simulink model "FSAC2021"  (R2014a)
settings: Solver=FixedStepDiscrete  StartTime=0.0  StopTime=inf  FixedStep=0.0005  RelTol=1e-3
model workspace (MAT data in the model file):
  MCOS : class17 (value not decoded)
  MCOS : class17 (value not decoded)
  MCOS : class17 (value not decoded)
  MCOS : class17 (value not decoded)
  MCOS : class17 (value not decoded)
  MCOS : class17 (value not decoded)
  MCOS : class17 (value not decoded)
  MCOS : class17 (value not decoded)
  MCOS : class17 (value not decoded)
  MCOS : class17 (value not decoded)
  MCOS : class17 (value not decoded)
  MCOS : class17 (value not decoded)
  MCOS : class17 (value not decoded)
  MCOS : class17 (value not decoded)
  MCOS : class17 (value not decoded)
  MCOS : class17 (value not decoded)
  MCOS : class17 (value not decoded)
  MCOS : class17 (value not decoded)
  MCOS : class17 (value not decoded)
  BUZZER_START = 1
  MCOS : class17 (value not decoded)
  MCOS : class17 (value not decoded)
  MCOS : class17 (value not decoded)
  MCOS : class17 (value not decoded)
  MCOS : class17 (value not decoded)
  MCOS : class17 (value not decoded)
  MCOS : class17 (value not decoded)
  MCOS : class17 (value not decoded)
  MCOS : class17 (value not decoded)
  MCOS : class17 (value not decoded)
  MCOS : class17 (value not decoded)
  MCOS : class17 (value not decoded)
  MCOS : class17 (value not decoded)
  MCOS : class17 (value not decoded)
  MCOS : class17 (value not decoded)
  MCOS : class17 (value not decoded)
  MCOS : class17 (value not decoded)
  MCOS : class17 (value not decoded)
  MCOS : class17 (value not decoded)
  MCOS : class17 (value not decoded)
  MCOS : class17 (value not decoded)
  MCOS : class17 (value not decoded)
  MCOS : class17 (value not decoded)
  MCOS : class17 (value not decoded)
  MCOS : class17 (value not decoded)
  MCOS : class17 (value not decoded)
  MCOS : class17 (value not decoded)
  MCOS : class17 (value not decoded)
  MCOS : class17 (value not decoded)
  MCOS : class17 (value not decoded)
  MCOS : class17 (value not decoded)
  MCOS : class17 (value not decoded)
  MCOS : class17 (value not decoded)
  MCOS : class17 (value not decoded)
  MCOS : class17 (value not decoded)
  MCOS : class17 (value not decoded)
  MCOS : class17 (value not decoded)
  MCOS : class17 (value not decoded)
  Brake = 11
  MCOS : class17 (value not decoded)
  MCOS : class17 (value not decoded)
  MCOS : class17 (value not decoded)
  MCOS : class17 (value not decoded)
  MCOS : class17 (value not decoded)
  MCOS : class17 (value not decoded)
  MCOS : class17 (value not decoded)
  MCOS : class17 (value not decoded)
  Sensor_Acc_b = 101.85
  Sensor_Acc_k = -0.0185
  Str_Sen_Orig_Angle = -341
  MCOS : class17 (value not decoded)
  Tire_D = 0.47
  T = 0.05
libraries: simulink x396, ec55xxlib x126
(part 13 of 17)

== system FSAC2021/ROUTING/TO_DCAN/Subsystem/DIAG_BCU/Brake_encoder_fault_sts ==
  Brake_encoder_fault_sts : Inport
  Brake_encoder_fault_stsRon : Rounding  Operator=round
  Brake_encoder_fault_sts_1sat : Saturate  UpperLimit=64  LowerLimit=0
  Brake_encoder_fault_sts_Convert : DataTypeConversion  OutDataTypeStr=uint8
  Brake_encoder_fault_sts_Convert1 : DataTypeConversion  OutDataTypeStr=uint32
  Brake_encoder_fault_sts_D : Product  Inputs=*/
  Brake_encoder_fault_sts_F : Constant  OutDataTypeStr=single
  Brake_encoder_fault_sts_L : simulink/Logic and Bit Operations/Bitwise Operator  logicop=AND  UseBitMask=on  BitMask=64  BitMaskRealWorld=Stored Integer
  Brake_encoder_fault_sts_O : Constant  Value=0  OutDataTypeStr=single
  Brake_encoder_fault_sts_S : ArithShift  BitShiftNumber=-6
  Brake_encoder_fault_sts_sat : Saturate  UpperLimit=1  LowerLimit=0
  Brake_encoder_fault_sts_st : Sum  Inputs=+-
  output4 : Outport
  wires:
  Brake_encoder_fault_sts/1 -> Brake_encoder_fault_sts_sat/1
  Brake_encoder_fault_sts_sat/1 -> Brake_encoder_fault_sts_st/1
  Brake_encoder_fault_sts_O/1 -> Brake_encoder_fault_sts_st/2
  Brake_encoder_fault_sts_st/1 -> Brake_encoder_fault_sts_D/1
  Brake_encoder_fault_sts_F/1 -> Brake_encoder_fault_sts_D/2
  Brake_encoder_fault_sts_D/1 -> Brake_encoder_fault_stsRon/1
  Brake_encoder_fault_stsRon/1 -> Brake_encoder_fault_sts_S/1
  Brake_encoder_fault_sts_S/1 -> Brake_encoder_fault_sts_1sat/1
  Brake_encoder_fault_sts_1sat/1 -> Brake_encoder_fault_sts_Convert1/1
  Brake_encoder_fault_sts_Convert1/1 -> Brake_encoder_fault_sts_L/1
  Brake_encoder_fault_sts_L/1 -> Brake_encoder_fault_sts_Convert/1
  Brake_encoder_fault_sts_Convert/1 -> output4/1

== system FSAC2021/ROUTING/TO_DCAN/Subsystem/DIAG_BCU/Brake_lowvolt_prtct_sts ==
  Brake_lowvolt_prtct_sts : Inport
  Brake_lowvolt_prtct_stsRon : Rounding  Operator=round
  Brake_lowvolt_prtct_sts_1sat : Saturate  UpperLimit=32  LowerLimit=0
  Brake_lowvolt_prtct_sts_Convert : DataTypeConversion  OutDataTypeStr=uint8
  Brake_lowvolt_prtct_sts_Convert1 : DataTypeConversion  OutDataTypeStr=uint32
  Brake_lowvolt_prtct_sts_D : Product  Inputs=*/
  Brake_lowvolt_prtct_sts_F : Constant  OutDataTypeStr=single
  Brake_lowvolt_prtct_sts_L : simulink/Logic and Bit Operations/Bitwise Operator  logicop=AND  UseBitMask=on  BitMask=32  BitMaskRealWorld=Stored Integer
  Brake_lowvolt_prtct_sts_O : Constant  Value=0  OutDataTypeStr=single
  Brake_lowvolt_prtct_sts_S : ArithShift  BitShiftNumber=-5
  Brake_lowvolt_prtct_sts_sat : Saturate  UpperLimit=1  LowerLimit=0
  Brake_lowvolt_prtct_sts_st : Sum  Inputs=+-
  output4 : Outport
  wires:
  Brake_lowvolt_prtct_sts/1 -> Brake_lowvolt_prtct_sts_sat/1
  Brake_lowvolt_prtct_sts_sat/1 -> Brake_lowvolt_prtct_sts_st/1
  Brake_lowvolt_prtct_sts_O/1 -> Brake_lowvolt_prtct_sts_st/2
  Brake_lowvolt_prtct_sts_st/1 -> Brake_lowvolt_prtct_sts_D/1
  Brake_lowvolt_prtct_sts_F/1 -> Brake_lowvolt_prtct_sts_D/2
  Brake_lowvolt_prtct_sts_D/1 -> Brake_lowvolt_prtct_stsRon/1
  Brake_lowvolt_prtct_stsRon/1 -> Brake_lowvolt_prtct_sts_S/1
  Brake_lowvolt_prtct_sts_S/1 -> Brake_lowvolt_prtct_sts_1sat/1
  Brake_lowvolt_prtct_sts_1sat/1 -> Brake_lowvolt_prtct_sts_Convert1/1
  Brake_lowvolt_prtct_sts_Convert1/1 -> Brake_lowvolt_prtct_sts_L/1
  Brake_lowvolt_prtct_sts_L/1 -> Brake_lowvolt_prtct_sts_Convert/1
  Brake_lowvolt_prtct_sts_Convert/1 -> output4/1

== system FSAC2021/ROUTING/TO_DCAN/Subsystem/DIAG_BCU/Brake_mtr_enable_flag ==
  Brake_mtr_enable_flag : Inport
  Brake_mtr_enable_flagRon : Rounding  Operator=round
  Brake_mtr_enable_flag_1sat : Saturate  UpperLimit=1  LowerLimit=0
  Brake_mtr_enable_flag_Convert : DataTypeConversion  OutDataTypeStr=uint8
  Brake_mtr_enable_flag_Convert1 : DataTypeConversion  OutDataTypeStr=uint32
  Brake_mtr_enable_flag_D : Product  Inputs=*/
  Brake_mtr_enable_flag_F : Constant  OutDataTypeStr=single
  Brake_mtr_enable_flag_L : simulink/Logic and Bit Operations/Bitwise Operator  logicop=AND  UseBitMask=on  BitMask=1  BitMaskRealWorld=Stored Integer
  Brake_mtr_enable_flag_O : Constant  Value=0  OutDataTypeStr=single
  Brake_mtr_enable_flag_S : ArithShift
  Brake_mtr_enable_flag_sat : Saturate  UpperLimit=1  LowerLimit=0
  Brake_mtr_enable_flag_st : Sum  Inputs=+-
  output4 : Outport
  wires:
  Brake_mtr_enable_flag/1 -> Brake_mtr_enable_flag_sat/1
  Brake_mtr_enable_flag_sat/1 -> Brake_mtr_enable_flag_st/1
  Brake_mtr_enable_flag_O/1 -> Brake_mtr_enable_flag_st/2
  Brake_mtr_enable_flag_st/1 -> Brake_mtr_enable_flag_D/1
  Brake_mtr_enable_flag_F/1 -> Brake_mtr_enable_flag_D/2
  Brake_mtr_enable_flag_D/1 -> Brake_mtr_enable_flagRon/1
  Brake_mtr_enable_flagRon/1 -> Brake_mtr_enable_flag_S/1
  Brake_mtr_enable_flag_S/1 -> Brake_mtr_enable_flag_1sat/1
  Brake_mtr_enable_flag_1sat/1 -> Brake_mtr_enable_flag_Convert1/1
  Brake_mtr_enable_flag_Convert1/1 -> Brake_mtr_enable_flag_L/1
  Brake_mtr_enable_flag_L/1 -> Brake_mtr_enable_flag_Convert/1
  Brake_mtr_enable_flag_Convert/1 -> output4/1

== system FSAC2021/ROUTING/TO_DCAN/Subsystem/DIAG_BCU/Brake_mtr_origin_flag ==
  Brake_mtr_origin_flag : Inport
  Brake_mtr_origin_flagRon : Rounding  Operator=round
  Brake_mtr_origin_flag_1sat : Saturate  UpperLimit=64  LowerLimit=0
  Brake_mtr_origin_flag_Convert : DataTypeConversion  OutDataTypeStr=uint8
  Brake_mtr_origin_flag_Convert1 : DataTypeConversion  OutDataTypeStr=uint32
  Brake_mtr_origin_flag_D : Product  Inputs=*/
  Brake_mtr_origin_flag_F : Constant  OutDataTypeStr=single
  Brake_mtr_origin_flag_L : simulink/Logic and Bit Operations/Bitwise Operator  logicop=AND  UseBitMask=on  BitMask=64  BitMaskRealWorld=Stored Integer
  Brake_mtr_origin_flag_O : Constant  Value=0  OutDataTypeStr=single
  Brake_mtr_origin_flag_S : ArithShift  BitShiftNumber=-6
  Brake_mtr_origin_flag_sat : Saturate  UpperLimit=1  LowerLimit=0
  Brake_mtr_origin_flag_st : Sum  Inputs=+-
  output3 : Outport
  wires:
  Brake_mtr_origin_flag/1 -> Brake_mtr_origin_flag_sat/1
  Brake_mtr_origin_flag_sat/1 -> Brake_mtr_origin_flag_st/1
  Brake_mtr_origin_flag_O/1 -> Brake_mtr_origin_flag_st/2
  Brake_mtr_origin_flag_st/1 -> Brake_mtr_origin_flag_D/1
  Brake_mtr_origin_flag_F/1 -> Brake_mtr_origin_flag_D/2
  Brake_mtr_origin_flag_D/1 -> Brake_mtr_origin_flagRon/1
  Brake_mtr_origin_flagRon/1 -> Brake_mtr_origin_flag_S/1
  Brake_mtr_origin_flag_S/1 -> Brake_mtr_origin_flag_1sat/1
  Brake_mtr_origin_flag_1sat/1 -> Brake_mtr_origin_flag_Convert1/1
  Brake_mtr_origin_flag_Convert1/1 -> Brake_mtr_origin_flag_L/1
  Brake_mtr_origin_flag_L/1 -> Brake_mtr_origin_flag_Convert/1
  Brake_mtr_origin_flag_Convert/1 -> output3/1

== system FSAC2021/ROUTING/TO_DCAN/Subsystem/DIAG_BCU/Brake_mtr_stop_flag ==
  Brake_mtr_stop_flag : Inport
  Brake_mtr_stop_flagRon : Rounding  Operator=round
  Brake_mtr_stop_flag_1sat : Saturate  UpperLimit=128  LowerLimit=0
  Brake_mtr_stop_flag_Convert : DataTypeConversion  OutDataTypeStr=uint8
  Brake_mtr_stop_flag_Convert1 : DataTypeConversion  OutDataTypeStr=uint32
  Brake_mtr_stop_flag_D : Product  Inputs=*/
  Brake_mtr_stop_flag_F : Constant  OutDataTypeStr=single
  Brake_mtr_stop_flag_L : simulink/Logic and Bit Operations/Bitwise Operator  logicop=AND  UseBitMask=on  BitMask=128  BitMaskRealWorld=Stored Integer
  Brake_mtr_stop_flag_O : Constant  Value=0  OutDataTypeStr=single
  Brake_mtr_stop_flag_S : ArithShift  BitShiftNumber=-7
  Brake_mtr_stop_flag_sat : Saturate  UpperLimit=1  LowerLimit=0
  Brake_mtr_stop_flag_st : Sum  Inputs=+-
  output3 : Outport
  wires:
  Brake_mtr_stop_flag/1 -> Brake_mtr_stop_flag_sat/1
  Brake_mtr_stop_flag_sat/1 -> Brake_mtr_stop_flag_st/1
  Brake_mtr_stop_flag_O/1 -> Brake_mtr_stop_flag_st/2
  Brake_mtr_stop_flag_st/1 -> Brake_mtr_stop_flag_D/1
  Brake_mtr_stop_flag_F/1 -> Brake_mtr_stop_flag_D/2
  Brake_mtr_stop_flag_D/1 -> Brake_mtr_stop_flagRon/1
  Brake_mtr_stop_flagRon/1 -> Brake_mtr_stop_flag_S/1
  Brake_mtr_stop_flag_S/1 -> Brake_mtr_stop_flag_1sat/1
  Brake_mtr_stop_flag_1sat/1 -> Brake_mtr_stop_flag_Convert1/1
  Brake_mtr_stop_flag_Convert1/1 -> Brake_mtr_stop_flag_L/1
  Brake_mtr_stop_flag_L/1 -> Brake_mtr_stop_flag_Convert/1
  Brake_mtr_stop_flag_Convert/1 -> output3/1

== system FSAC2021/ROUTING/TO_DCAN/Subsystem/DIAG_BCU/Brake_overcurrt_prtct_sts ==
  Brake_overcurrt_prtct_sts : Inport
  Brake_overcurrt_prtct_stsRon : Rounding  Operator=round
  Brake_overcurrt_prtct_sts_1sat : Saturate  UpperLimit=16  LowerLimit=0
  Brake_overcurrt_prtct_sts_Convert : DataTypeConversion  OutDataTypeStr=uint8
  Brake_overcurrt_prtct_sts_Convert1 : DataTypeConversion  OutDataTypeStr=uint32
  Brake_overcurrt_prtct_sts_D : Product  Inputs=*/
  Brake_overcurrt_prtct_sts_F : Constant  OutDataTypeStr=single
  Brake_overcurrt_prtct_sts_L : simulink/Logic and Bit Operations/Bitwise Operator  logicop=AND  UseBitMask=on  BitMask=16  BitMaskRealWorld=Stored Integer
  Brake_overcurrt_prtct_sts_O : Constant  Value=0  OutDataTypeStr=single
  Brake_overcurrt_prtct_sts_S : ArithShift  BitShiftNumber=-4
  Brake_overcurrt_prtct_sts_sat : Saturate  UpperLimit=1  LowerLimit=0
  Brake_overcurrt_prtct_sts_st : Sum  Inputs=+-
  output4 : Outport
  wires:
  Brake_overcurrt_prtct_sts/1 -> Brake_overcurrt_prtct_sts_sat/1
  Brake_overcurrt_prtct_sts_sat/1 -> Brake_overcurrt_prtct_sts_st/1
  Brake_overcurrt_prtct_sts_O/1 -> Brake_overcurrt_prtct_sts_st/2
  Brake_overcurrt_prtct_sts_st/1 -> Brake_overcurrt_prtct_sts_D/1
  Brake_overcurrt_prtct_sts_F/1 -> Brake_overcurrt_prtct_sts_D/2
  Brake_overcurrt_prtct_sts_D/1 -> Brake_overcurrt_prtct_stsRon/1
  Brake_overcurrt_prtct_stsRon/1 -> Brake_overcurrt_prtct_sts_S/1
  Brake_overcurrt_prtct_sts_S/1 -> Brake_overcurrt_prtct_sts_1sat/1
  Brake_overcurrt_prtct_sts_1sat/1 -> Brake_overcurrt_prtct_sts_Convert1/1
  Brake_overcurrt_prtct_sts_Convert1/1 -> Brake_overcurrt_prtct_sts_L/1
  Brake_overcurrt_prtct_sts_L/1 -> Brake_overcurrt_prtct_sts_Convert/1
  Brake_overcurrt_prtct_sts_Convert/1 -> output4/1

== system FSAC2021/ROUTING/TO_DCAN/Subsystem/DIAG_BCU/Brake_overheat_prtct_sts ==
  Brake_overheat_prtct_sts : Inport
  Brake_overheat_prtct_stsRon : Rounding  Operator=round
  Brake_overheat_prtct_sts_1sat : Saturate  UpperLimit=8  LowerLimit=0
  Brake_overheat_prtct_sts_Convert : DataTypeConversion  OutDataTypeStr=uint8
  Brake_overheat_prtct_sts_Convert1 : DataTypeConversion  OutDataTypeStr=uint32
  Brake_overheat_prtct_sts_D : Product  Inputs=*/
  Brake_overheat_prtct_sts_F : Constant  OutDataTypeStr=single
  Brake_overheat_prtct_sts_L : simulink/Logic and Bit Operations/Bitwise Operator  logicop=AND  UseBitMask=on  BitMask=8  BitMaskRealWorld=Stored Integer
  Brake_overheat_prtct_sts_O : Constant  Value=0  OutDataTypeStr=single
  Brake_overheat_prtct_sts_S : ArithShift  BitShiftNumber=-3
  Brake_overheat_prtct_sts_sat : Saturate  UpperLimit=1  LowerLimit=0
  Brake_overheat_prtct_sts_st : Sum  Inputs=+-
  output4 : Outport
  wires:
  Brake_overheat_prtct_sts/1 -> Brake_overheat_prtct_sts_sat/1
  Brake_overheat_prtct_sts_sat/1 -> Brake_overheat_prtct_sts_st/1
  Brake_overheat_prtct_sts_O/1 -> Brake_overheat_prtct_sts_st/2
  Brake_overheat_prtct_sts_st/1 -> Brake_overheat_prtct_sts_D/1
  Brake_overheat_prtct_sts_F/1 -> Brake_overheat_prtct_sts_D/2
  Brake_overheat_prtct_sts_D/1 -> Brake_overheat_prtct_stsRon/1
  Brake_overheat_prtct_stsRon/1 -> Brake_overheat_prtct_sts_S/1
  Brake_overheat_prtct_sts_S/1 -> Brake_overheat_prtct_sts_1sat/1
  Brake_overheat_prtct_sts_1sat/1 -> Brake_overheat_prtct_sts_Convert1/1
  Brake_overheat_prtct_sts_Convert1/1 -> Brake_overheat_prtct_sts_L/1
  Brake_overheat_prtct_sts_L/1 -> Brake_overheat_prtct_sts_Convert/1
  Brake_overheat_prtct_sts_Convert/1 -> output4/1

== system FSAC2021/ROUTING/TO_DCAN/Subsystem/DIAG_BCU/Brake_reg_rw_fault_flag ==
  Brake_reg_rw_fault_flag : Inport
  Brake_reg_rw_fault_flagRon : Rounding  Operator=round
  Brake_reg_rw_fault_flag_1sat : Saturate  UpperLimit=2  LowerLimit=0
  Brake_reg_rw_fault_flag_Convert : DataTypeConversion  OutDataTypeStr=uint8
  Brake_reg_rw_fault_flag_Convert1 : DataTypeConversion  OutDataTypeStr=uint32
  Brake_reg_rw_fault_flag_D : Product  Inputs=*/
  Brake_reg_rw_fault_flag_F : Constant  OutDataTypeStr=single
  Brake_reg_rw_fault_flag_L : simulink/Logic and Bit Operations/Bitwise Operator  logicop=AND  UseBitMask=on  BitMask=2  BitMaskRealWorld=Stored Integer
  Brake_reg_rw_fault_flag_O : Constant  Value=0  OutDataTypeStr=single
  Brake_reg_rw_fault_flag_S : ArithShift  BitShiftNumber=-1
  Brake_reg_rw_fault_flag_sat : Saturate  UpperLimit=1  LowerLimit=0
  Brake_reg_rw_fault_flag_st : Sum  Inputs=+-
  output4 : Outport
  wires:
  Brake_reg_rw_fault_flag/1 -> Brake_reg_rw_fault_flag_sat/1
  Brake_reg_rw_fault_flag_sat/1 -> Brake_reg_rw_fault_flag_st/1
  Brake_reg_rw_fault_flag_O/1 -> Brake_reg_rw_fault_flag_st/2
  Brake_reg_rw_fault_flag_st/1 -> Brake_reg_rw_fault_flag_D/1
  Brake_reg_rw_fault_flag_F/1 -> Brake_reg_rw_fault_flag_D/2
  Brake_reg_rw_fault_flag_D/1 -> Brake_reg_rw_fault_flagRon/1
  Brake_reg_rw_fault_flagRon/1 -> Brake_reg_rw_fault_flag_S/1
  Brake_reg_rw_fault_flag_S/1 -> Brake_reg_rw_fault_flag_1sat/1
  Brake_reg_rw_fault_flag_1sat/1 -> Brake_reg_rw_fault_flag_Convert1/1
  Brake_reg_rw_fault_flag_Convert1/1 -> Brake_reg_rw_fault_flag_L/1
  Brake_reg_rw_fault_flag_L/1 -> Brake_reg_rw_fault_flag_Convert/1
  Brake_reg_rw_fault_flag_Convert/1 -> output4/1

== system FSAC2021/ROUTING/TO_DCAN/Subsystem/DIAG_BCU/Brake_sensor1_sts ==
  Brake_sensor1_sts : Inport
  Brake_sensor1_stsRon : Rounding  Operator=round
  Brake_sensor1_sts_1sat : Saturate  UpperLimit=1  LowerLimit=0
  Brake_sensor1_sts_Convert : DataTypeConversion  OutDataTypeStr=uint8
  Brake_sensor1_sts_Convert1 : DataTypeConversion  OutDataTypeStr=uint32
  Brake_sensor1_sts_D : Product  Inputs=*/
  Brake_sensor1_sts_F : Constant  OutDataTypeStr=single
  Brake_sensor1_sts_L : simulink/Logic and Bit Operations/Bitwise Operator  logicop=AND  UseBitMask=on  BitMask=1  BitMaskRealWorld=Stored Integer
  Brake_sensor1_sts_O : Constant  Value=0  OutDataTypeStr=single
  Brake_sensor1_sts_S : ArithShift
  Brake_sensor1_sts_sat : Saturate  UpperLimit=1  LowerLimit=0
  Brake_sensor1_sts_st : Sum  Inputs=+-
  output3 : Outport
  wires:
  Brake_sensor1_sts/1 -> Brake_sensor1_sts_sat/1
  Brake_sensor1_sts_sat/1 -> Brake_sensor1_sts_st/1
  Brake_sensor1_sts_O/1 -> Brake_sensor1_sts_st/2
  Brake_sensor1_sts_st/1 -> Brake_sensor1_sts_D/1
  Brake_sensor1_sts_F/1 -> Brake_sensor1_sts_D/2
  Brake_sensor1_sts_D/1 -> Brake_sensor1_stsRon/1
  Brake_sensor1_stsRon/1 -> Brake_sensor1_sts_S/1
  Brake_sensor1_sts_S/1 -> Brake_sensor1_sts_1sat/1
  Brake_sensor1_sts_1sat/1 -> Brake_sensor1_sts_Convert1/1
  Brake_sensor1_sts_Convert1/1 -> Brake_sensor1_sts_L/1
  Brake_sensor1_sts_L/1 -> Brake_sensor1_sts_Convert/1
  Brake_sensor1_sts_Convert/1 -> output3/1

== system FSAC2021/ROUTING/TO_DCAN/Subsystem/DIAG_BCU/Brake_sensor2_sts ==
  Brake_sensor2_sts : Inport
  Brake_sensor2_stsRon : Rounding  Operator=round
  Brake_sensor2_sts_1sat : Saturate  UpperLimit=2  LowerLimit=0
  Brake_sensor2_sts_Convert : DataTypeConversion  OutDataTypeStr=uint8
  Brake_sensor2_sts_Convert1 : DataTypeConversion  OutDataTypeStr=uint32
  Brake_sensor2_sts_D : Product  Inputs=*/
  Brake_sensor2_sts_F : Constant  OutDataTypeStr=single
  Brake_sensor2_sts_L : simulink/Logic and Bit Operations/Bitwise Operator  logicop=AND  UseBitMask=on  BitMask=2  BitMaskRealWorld=Stored Integer
  Brake_sensor2_sts_O : Constant  Value=0  OutDataTypeStr=single
  Brake_sensor2_sts_S : ArithShift  BitShiftNumber=-1
  Brake_sensor2_sts_sat : Saturate  UpperLimit=1  LowerLimit=0
  Brake_sensor2_sts_st : Sum  Inputs=+-
  output3 : Outport
  wires:
  Brake_sensor2_sts/1 -> Brake_sensor2_sts_sat/1
  Brake_sensor2_sts_sat/1 -> Brake_sensor2_sts_st/1
  Brake_sensor2_sts_O/1 -> Brake_sensor2_sts_st/2
  Brake_sensor2_sts_st/1 -> Brake_sensor2_sts_D/1
  Brake_sensor2_sts_F/1 -> Brake_sensor2_sts_D/2
  Brake_sensor2_sts_D/1 -> Brake_sensor2_stsRon/1
  Brake_sensor2_stsRon/1 -> Brake_sensor2_sts_S/1
  Brake_sensor2_sts_S/1 -> Brake_sensor2_sts_1sat/1
  Brake_sensor2_sts_1sat/1 -> Brake_sensor2_sts_Convert1/1
  Brake_sensor2_sts_Convert1/1 -> Brake_sensor2_sts_L/1
  Brake_sensor2_sts_L/1 -> Brake_sensor2_sts_Convert/1
  Brake_sensor2_sts_Convert/1 -> output3/1

== system FSAC2021/ROUTING/TO_DCAN/Subsystem/DIAG_BCU/Brake_sensor3_sts ==
  Brake_sensor3_sts : Inport
  Brake_sensor3_stsRon : Rounding  Operator=round
  Brake_sensor3_sts_1sat : Saturate  UpperLimit=4  LowerLimit=0
  Brake_sensor3_sts_Convert : DataTypeConversion  OutDataTypeStr=uint8
  Brake_sensor3_sts_Convert1 : DataTypeConversion  OutDataTypeStr=uint32
  Brake_sensor3_sts_D : Product  Inputs=*/
  Brake_sensor3_sts_F : Constant  OutDataTypeStr=single
  Brake_sensor3_sts_L : simulink/Logic and Bit Operations/Bitwise Operator  logicop=AND  UseBitMask=on  BitMask=4  BitMaskRealWorld=Stored Integer
  Brake_sensor3_sts_O : Constant  Value=0  OutDataTypeStr=single
  Brake_sensor3_sts_S : ArithShift  BitShiftNumber=-2
  Brake_sensor3_sts_sat : Saturate  UpperLimit=1  LowerLimit=0
  Brake_sensor3_sts_st : Sum  Inputs=+-
  output3 : Outport
  wires:
  Brake_sensor3_sts/1 -> Brake_sensor3_sts_sat/1
  Brake_sensor3_sts_sat/1 -> Brake_sensor3_sts_st/1
  Brake_sensor3_sts_O/1 -> Brake_sensor3_sts_st/2
  Brake_sensor3_sts_st/1 -> Brake_sensor3_sts_D/1
  Brake_sensor3_sts_F/1 -> Brake_sensor3_sts_D/2
  Brake_sensor3_sts_D/1 -> Brake_sensor3_stsRon/1
  Brake_sensor3_stsRon/1 -> Brake_sensor3_sts_S/1
  Brake_sensor3_sts_S/1 -> Brake_sensor3_sts_1sat/1
  Brake_sensor3_sts_1sat/1 -> Brake_sensor3_sts_Convert1/1
  Brake_sensor3_sts_Convert1/1 -> Brake_sensor3_sts_L/1
  Brake_sensor3_sts_L/1 -> Brake_sensor3_sts_Convert/1
  Brake_sensor3_sts_Convert/1 -> output3/1

== system FSAC2021/ROUTING/TO_DCAN/Subsystem/DIAG_BCU/Brake_sensor4_sts ==
  Brake_sensor4_sts : Inport
  Brake_sensor4_stsRon : Rounding  Operator=round
  Brake_sensor4_sts_1sat : Saturate  UpperLimit=8  LowerLimit=0
  Brake_sensor4_sts_Convert : DataTypeConversion  OutDataTypeStr=uint8
  Brake_sensor4_sts_Convert1 : DataTypeConversion  OutDataTypeStr=uint32
  Brake_sensor4_sts_D : Product  Inputs=*/
  Brake_sensor4_sts_F : Constant  OutDataTypeStr=single
  Brake_sensor4_sts_L : simulink/Logic and Bit Operations/Bitwise Operator  logicop=AND  UseBitMask=on  BitMask=8  BitMaskRealWorld=Stored Integer
  Brake_sensor4_sts_O : Constant  Value=0  OutDataTypeStr=single
  Brake_sensor4_sts_S : ArithShift  BitShiftNumber=-3
  Brake_sensor4_sts_sat : Saturate  UpperLimit=1  LowerLimit=0
  Brake_sensor4_sts_st : Sum  Inputs=+-
  output3 : Outport
  wires:
  Brake_sensor4_sts/1 -> Brake_sensor4_sts_sat/1
  Brake_sensor4_sts_sat/1 -> Brake_sensor4_sts_st/1
  Brake_sensor4_sts_O/1 -> Brake_sensor4_sts_st/2
  Brake_sensor4_sts_st/1 -> Brake_sensor4_sts_D/1
  Brake_sensor4_sts_F/1 -> Brake_sensor4_sts_D/2
  Brake_sensor4_sts_D/1 -> Brake_sensor4_stsRon/1
  Brake_sensor4_stsRon/1 -> Brake_sensor4_sts_S/1
  Brake_sensor4_sts_S/1 -> Brake_sensor4_sts_1sat/1
  Brake_sensor4_sts_1sat/1 -> Brake_sensor4_sts_Convert1/1
  Brake_sensor4_sts_Convert1/1 -> Brake_sensor4_sts_L/1
  Brake_sensor4_sts_L/1 -> Brake_sensor4_sts_Convert/1
  Brake_sensor4_sts_Convert/1 -> output3/1

== system FSAC2021/ROUTING/TO_DCAN/Subsystem/DIAG_BCU/Brake_sensor5_sts ==
  Brake_sensor5_sts : Inport
  Brake_sensor5_stsRon : Rounding  Operator=round
  Brake_sensor5_sts_1sat : Saturate  UpperLimit=16  LowerLimit=0
  Brake_sensor5_sts_Convert : DataTypeConversion  OutDataTypeStr=uint8
  Brake_sensor5_sts_Convert1 : DataTypeConversion  OutDataTypeStr=uint32
  Brake_sensor5_sts_D : Product  Inputs=*/
  Brake_sensor5_sts_F : Constant  OutDataTypeStr=single
  Brake_sensor5_sts_L : simulink/Logic and Bit Operations/Bitwise Operator  logicop=AND  UseBitMask=on  BitMask=16  BitMaskRealWorld=Stored Integer
  Brake_sensor5_sts_O : Constant  Value=0  OutDataTypeStr=single
  Brake_sensor5_sts_S : ArithShift  BitShiftNumber=-4
  Brake_sensor5_sts_sat : Saturate  UpperLimit=1  LowerLimit=0
  Brake_sensor5_sts_st : Sum  Inputs=+-
  output3 : Outport
  wires:
  Brake_sensor5_sts/1 -> Brake_sensor5_sts_sat/1
  Brake_sensor5_sts_sat/1 -> Brake_sensor5_sts_st/1
  Brake_sensor5_sts_O/1 -> Brake_sensor5_sts_st/2
  Brake_sensor5_sts_st/1 -> Brake_sensor5_sts_D/1
  Brake_sensor5_sts_F/1 -> Brake_sensor5_sts_D/2
  Brake_sensor5_sts_D/1 -> Brake_sensor5_stsRon/1
  Brake_sensor5_stsRon/1 -> Brake_sensor5_sts_S/1
  Brake_sensor5_sts_S/1 -> Brake_sensor5_sts_1sat/1
  Brake_sensor5_sts_1sat/1 -> Brake_sensor5_sts_Convert1/1
  Brake_sensor5_sts_Convert1/1 -> Brake_sensor5_sts_L/1
  Brake_sensor5_sts_L/1 -> Brake_sensor5_sts_Convert/1
  Brake_sensor5_sts_Convert/1 -> output3/1

== system FSAC2021/ROUTING/TO_DCAN/Subsystem/DIAG_BCU/Brake_sensor6_sts ==
  Brake_sensor6_sts : Inport
  Brake_sensor6_stsRon : Rounding  Operator=round
  Brake_sensor6_sts_1sat : Saturate  UpperLimit=32  LowerLimit=0
  Brake_sensor6_sts_Convert : DataTypeConversion  OutDataTypeStr=uint8
  Brake_sensor6_sts_Convert1 : DataTypeConversion  OutDataTypeStr=uint32
  Brake_sensor6_sts_D : Product  Inputs=*/
  Brake_sensor6_sts_F : Constant  OutDataTypeStr=single
  Brake_sensor6_sts_L : simulink/Logic and Bit Operations/Bitwise Operator  logicop=AND  UseBitMask=on  BitMask=32  BitMaskRealWorld=Stored Integer
  Brake_sensor6_sts_O : Constant  Value=0  OutDataTypeStr=single
  Brake_sensor6_sts_S : ArithShift  BitShiftNumber=-5
  Brake_sensor6_sts_sat : Saturate  UpperLimit=1  LowerLimit=0
  Brake_sensor6_sts_st : Sum  Inputs=+-
  output3 : Outport
  wires:
  Brake_sensor6_sts/1 -> Brake_sensor6_sts_sat/1
  Brake_sensor6_sts_sat/1 -> Brake_sensor6_sts_st/1
  Brake_sensor6_sts_O/1 -> Brake_sensor6_sts_st/2
  Brake_sensor6_sts_st/1 -> Brake_sensor6_sts_D/1
  Brake_sensor6_sts_F/1 -> Brake_sensor6_sts_D/2
  Brake_sensor6_sts_D/1 -> Brake_sensor6_stsRon/1
  Brake_sensor6_stsRon/1 -> Brake_sensor6_sts_S/1
  Brake_sensor6_sts_S/1 -> Brake_sensor6_sts_1sat/1
  Brake_sensor6_sts_1sat/1 -> Brake_sensor6_sts_Convert1/1
  Brake_sensor6_sts_Convert1/1 -> Brake_sensor6_sts_L/1
  Brake_sensor6_sts_L/1 -> Brake_sensor6_sts_Convert/1
  Brake_sensor6_sts_Convert/1 -> output3/1

== system FSAC2021/ROUTING/TO_DCAN/Subsystem/DIAG_BMS_ALARM_RELAY/ALM_AUX_FAIL ==
  ALM_AUX_FAIL : Inport
  ALM_AUX_FAILRon : Rounding  Operator=round
  ALM_AUX_FAIL_1sat : Saturate  UpperLimit=16  LowerLimit=0
  ALM_AUX_FAIL_Convert : DataTypeConversion  OutDataTypeStr=uint8
  ALM_AUX_FAIL_Convert1 : DataTypeConversion  OutDataTypeStr=uint32
  ALM_AUX_FAIL_D : Product  Inputs=*/
  ALM_AUX_FAIL_F : Constant  OutDataTypeStr=single
  ALM_AUX_FAIL_L : simulink/Logic and Bit Operations/Bitwise Operator  logicop=AND  UseBitMask=on  BitMask=16  BitMaskRealWorld=Stored Integer
  ALM_AUX_FAIL_O : Constant  Value=0  OutDataTypeStr=single
  ALM_AUX_FAIL_S : ArithShift  BitShiftNumber=-4
  ALM_AUX_FAIL_sat : Saturate  UpperLimit=1  LowerLimit=0
  ALM_AUX_FAIL_st : Sum  Inputs=+-
  output3 : Outport
  wires:
  ALM_AUX_FAIL/1 -> ALM_AUX_FAIL_sat/1
  ALM_AUX_FAIL_sat/1 -> ALM_AUX_FAIL_st/1
  ALM_AUX_FAIL_O/1 -> ALM_AUX_FAIL_st/2
  ALM_AUX_FAIL_st/1 -> ALM_AUX_FAIL_D/1
  ALM_AUX_FAIL_F/1 -> ALM_AUX_FAIL_D/2
  ALM_AUX_FAIL_D/1 -> ALM_AUX_FAILRon/1
  ALM_AUX_FAILRon/1 -> ALM_AUX_FAIL_S/1
  ALM_AUX_FAIL_S/1 -> ALM_AUX_FAIL_1sat/1
  ALM_AUX_FAIL_1sat/1 -> ALM_AUX_FAIL_Convert1/1
  ALM_AUX_FAIL_Convert1/1 -> ALM_AUX_FAIL_L/1
  ALM_AUX_FAIL_L/1 -> ALM_AUX_FAIL_Convert/1
  ALM_AUX_FAIL_Convert/1 -> output3/1

== system FSAC2021/ROUTING/TO_DCAN/Subsystem/DIAG_BMS_ALARM_RELAY/ALM_BATT_DT ==
  ALM_BATT_DT : Inport
  ALM_BATT_DTRon : Rounding  Operator=round
  ALM_BATT_DT_1sat : Saturate  UpperLimit=128  LowerLimit=0
  ALM_BATT_DT_Convert : DataTypeConversion  OutDataTypeStr=uint8
  ALM_BATT_DT_Convert1 : DataTypeConversion  OutDataTypeStr=uint32
  ALM_BATT_DT_D : Product  Inputs=*/
  ALM_BATT_DT_F : Constant  OutDataTypeStr=single
  ALM_BATT_DT_L : simulink/Logic and Bit Operations/Bitwise Operator  logicop=AND  UseBitMask=on  BitMask=128  BitMaskRealWorld=Stored Integer
  ALM_BATT_DT_O : Constant  Value=0  OutDataTypeStr=single
  ALM_BATT_DT_S : ArithShift  BitShiftNumber=-7
  ALM_BATT_DT_sat : Saturate  UpperLimit=1  LowerLimit=0
  ALM_BATT_DT_st : Sum  Inputs=+-
  output1 : Outport
  wires:
  ALM_BATT_DT/1 -> ALM_BATT_DT_sat/1
  ALM_BATT_DT_sat/1 -> ALM_BATT_DT_st/1
  ALM_BATT_DT_O/1 -> ALM_BATT_DT_st/2
  ALM_BATT_DT_st/1 -> ALM_BATT_DT_D/1
  ALM_BATT_DT_F/1 -> ALM_BATT_DT_D/2
  ALM_BATT_DT_D/1 -> ALM_BATT_DTRon/1
  ALM_BATT_DTRon/1 -> ALM_BATT_DT_S/1
  ALM_BATT_DT_S/1 -> ALM_BATT_DT_1sat/1
  ALM_BATT_DT_1sat/1 -> ALM_BATT_DT_Convert1/1
  ALM_BATT_DT_Convert1/1 -> ALM_BATT_DT_L/1
  ALM_BATT_DT_L/1 -> ALM_BATT_DT_Convert/1
  ALM_BATT_DT_Convert/1 -> output1/1

== system FSAC2021/ROUTING/TO_DCAN/Subsystem/DIAG_BMS_ALARM_RELAY/ALM_BATT_DV ==
  ALM_BATT_DV : Inport
  ALM_BATT_DVRon : Rounding  Operator=round
  ALM_BATT_DV_1sat : Saturate  UpperLimit=64  LowerLimit=0
  ALM_BATT_DV_Convert : DataTypeConversion  OutDataTypeStr=uint8
  ALM_BATT_DV_Convert1 : DataTypeConversion  OutDataTypeStr=uint32
  ALM_BATT_DV_D : Product  Inputs=*/
  ALM_BATT_DV_F : Constant  OutDataTypeStr=single
  ALM_BATT_DV_L : simulink/Logic and Bit Operations/Bitwise Operator  logicop=AND  UseBitMask=on  BitMask=64  BitMaskRealWorld=Stored Integer
  ALM_BATT_DV_O : Constant  Value=0  OutDataTypeStr=single
  ALM_BATT_DV_S : ArithShift  BitShiftNumber=-6
  ALM_BATT_DV_sat : Saturate  UpperLimit=1  LowerLimit=0
  ALM_BATT_DV_st : Sum  Inputs=+-
  output1 : Outport
  wires:
  ALM_BATT_DV/1 -> ALM_BATT_DV_sat/1
  ALM_BATT_DV_sat/1 -> ALM_BATT_DV_st/1
  ALM_BATT_DV_O/1 -> ALM_BATT_DV_st/2
  ALM_BATT_DV_st/1 -> ALM_BATT_DV_D/1
  ALM_BATT_DV_F/1 -> ALM_BATT_DV_D/2
  ALM_BATT_DV_D/1 -> ALM_BATT_DVRon/1
  ALM_BATT_DVRon/1 -> ALM_BATT_DV_S/1
  ALM_BATT_DV_S/1 -> ALM_BATT_DV_1sat/1
  ALM_BATT_DV_1sat/1 -> ALM_BATT_DV_Convert1/1
  ALM_BATT_DV_Convert1/1 -> ALM_BATT_DV_L/1
  ALM_BATT_DV_L/1 -> ALM_BATT_DV_Convert/1
  ALM_BATT_DV_Convert/1 -> output1/1

== system FSAC2021/ROUTING/TO_DCAN/Subsystem/DIAG_BMS_ALARM_RELAY/ALM_BATT_OC ==
  ALM_BATT_OC : Inport
  ALM_BATT_OCRon : Rounding  Operator=round
  ALM_BATT_OC_1sat : Saturate  UpperLimit=4  LowerLimit=0
  ALM_BATT_OC_Convert : DataTypeConversion  OutDataTypeStr=uint8
  ALM_BATT_OC_Convert1 : DataTypeConversion  OutDataTypeStr=uint32
  ALM_BATT_OC_D : Product  Inputs=*/
  ALM_BATT_OC_F : Constant  OutDataTypeStr=single
  ALM_BATT_OC_L : simulink/Logic and Bit Operations/Bitwise Operator  logicop=AND  UseBitMask=on  BitMask=4  BitMaskRealWorld=Stored Integer
  ALM_BATT_OC_O : Constant  Value=0  OutDataTypeStr=single
  ALM_BATT_OC_S : ArithShift  BitShiftNumber=-2
  ALM_BATT_OC_sat : Saturate  UpperLimit=1  LowerLimit=0
  ALM_BATT_OC_st : Sum  Inputs=+-
  output2 : Outport
  wires:
  ALM_BATT_OC/1 -> ALM_BATT_OC_sat/1
  ALM_BATT_OC_sat/1 -> ALM_BATT_OC_st/1
  ALM_BATT_OC_O/1 -> ALM_BATT_OC_st/2
  ALM_BATT_OC_st/1 -> ALM_BATT_OC_D/1
  ALM_BATT_OC_F/1 -> ALM_BATT_OC_D/2
  ALM_BATT_OC_D/1 -> ALM_BATT_OCRon/1
  ALM_BATT_OCRon/1 -> ALM_BATT_OC_S/1
  ALM_BATT_OC_S/1 -> ALM_BATT_OC_1sat/1
  ALM_BATT_OC_1sat/1 -> ALM_BATT_OC_Convert1/1
  ALM_BATT_OC_Convert1/1 -> ALM_BATT_OC_L/1
  ALM_BATT_OC_L/1 -> ALM_BATT_OC_Convert/1
  ALM_BATT_OC_Convert/1 -> output2/1

== system FSAC2021/ROUTING/TO_DCAN/Subsystem/DIAG_BMS_ALARM_RELAY/ALM_BATT_OV ==
  ALM_BATT_OV : Inport
  ALM_BATT_OVRon : Rounding  Operator=round
  ALM_BATT_OV_1sat : Saturate  UpperLimit=2  LowerLimit=0
  ALM_BATT_OV_Convert : DataTypeConversion  OutDataTypeStr=uint8
  ALM_BATT_OV_Convert1 : DataTypeConversion  OutDataTypeStr=uint32
  ALM_BATT_OV_D : Product  Inputs=*/
  ALM_BATT_OV_F : Constant  OutDataTypeStr=single
  ALM_BATT_OV_L : simulink/Logic and Bit Operations/Bitwise Operator  logicop=AND  UseBitMask=on  BitMask=2  BitMaskRealWorld=Stored Integer
  ALM_BATT_OV_O : Constant  Value=0  OutDataTypeStr=single
  ALM_BATT_OV_S : ArithShift  BitShiftNumber=-1
  ALM_BATT_OV_sat : Saturate  UpperLimit=1  LowerLimit=0
  ALM_BATT_OV_st : Sum  Inputs=+-
  output2 : Outport
  wires:
  ALM_BATT_OV/1 -> ALM_BATT_OV_sat/1
  ALM_BATT_OV_sat/1 -> ALM_BATT_OV_st/1
  ALM_BATT_OV_O/1 -> ALM_BATT_OV_st/2
  ALM_BATT_OV_st/1 -> ALM_BATT_OV_D/1
  ALM_BATT_OV_F/1 -> ALM_BATT_OV_D/2
  ALM_BATT_OV_D/1 -> ALM_BATT_OVRon/1
  ALM_BATT_OVRon/1 -> ALM_BATT_OV_S/1
  ALM_BATT_OV_S/1 -> ALM_BATT_OV_1sat/1
  ALM_BATT_OV_1sat/1 -> ALM_BATT_OV_Convert1/1
  ALM_BATT_OV_Convert1/1 -> ALM_BATT_OV_L/1
  ALM_BATT_OV_L/1 -> ALM_BATT_OV_Convert/1
  ALM_BATT_OV_Convert/1 -> output2/1

== system FSAC2021/ROUTING/TO_DCAN/Subsystem/DIAG_BMS_ALARM_RELAY/ALM_BATT_UC ==
  ALM_BATT_UC : Inport
  ALM_BATT_UCRon : Rounding  Operator=round
  ALM_BATT_UC_1sat : Saturate  UpperLimit=8  LowerLimit=0
  ALM_BATT_UC_Convert : DataTypeConversion  OutDataTypeStr=uint8
  ALM_BATT_UC_Convert1 : DataTypeConversion  OutDataTypeStr=uint32
  ALM_BATT_UC_D : Product  Inputs=*/
  ALM_BATT_UC_F : Constant  OutDataTypeStr=single
  ALM_BATT_UC_L : simulink/Logic and Bit Operations/Bitwise Operator  logicop=AND  UseBitMask=on  BitMask=8  BitMaskRealWorld=Stored Integer
  ALM_BATT_UC_O : Constant  Value=0  OutDataTypeStr=single
  ALM_BATT_UC_S : ArithShift  BitShiftNumber=-3
  ALM_BATT_UC_sat : Saturate  UpperLimit=1  LowerLimit=0
  ALM_BATT_UC_st : Sum  Inputs=+-
  output2 : Outport
  wires:
  ALM_BATT_UC/1 -> ALM_BATT_UC_sat/1
  ALM_BATT_UC_sat/1 -> ALM_BATT_UC_st/1
  ALM_BATT_UC_O/1 -> ALM_BATT_UC_st/2
  ALM_BATT_UC_st/1 -> ALM_BATT_UC_D/1
  ALM_BATT_UC_F/1 -> ALM_BATT_UC_D/2
  ALM_BATT_UC_D/1 -> ALM_BATT_UCRon/1
  ALM_BATT_UCRon/1 -> ALM_BATT_UC_S/1
  ALM_BATT_UC_S/1 -> ALM_BATT_UC_1sat/1
  ALM_BATT_UC_1sat/1 -> ALM_BATT_UC_Convert1/1
  ALM_BATT_UC_Convert1/1 -> ALM_BATT_UC_L/1
  ALM_BATT_UC_L/1 -> ALM_BATT_UC_Convert/1
  ALM_BATT_UC_Convert/1 -> output2/1

== system FSAC2021/ROUTING/TO_DCAN/Subsystem/DIAG_BMS_ALARM_RELAY/ALM_BATT_UV ==
  ALM_BATT_UV : Inport
  ALM_BATT_UVRon : Rounding  Operator=round
  ALM_BATT_UV_1sat : Saturate  UpperLimit=1  LowerLimit=0
  ALM_BATT_UV_Convert : DataTypeConversion  OutDataTypeStr=uint8
  ALM_BATT_UV_Convert1 : DataTypeConversion  OutDataTypeStr=uint32
  ALM_BATT_UV_D : Product  Inputs=*/
  ALM_BATT_UV_F : Constant  OutDataTypeStr=single
  ALM_BATT_UV_L : simulink/Logic and Bit Operations/Bitwise Operator  logicop=AND  UseBitMask=on  BitMask=1  BitMaskRealWorld=Stored Integer
  ALM_BATT_UV_O : Constant  Value=0  OutDataTypeStr=single
  ALM_BATT_UV_S : ArithShift
  ALM_BATT_UV_sat : Saturate  UpperLimit=1  LowerLimit=0
  ALM_BATT_UV_st : Sum  Inputs=+-
  output2 : Outport
  wires:
  ALM_BATT_UV/1 -> ALM_BATT_UV_sat/1
  ALM_BATT_UV_sat/1 -> ALM_BATT_UV_st/1
  ALM_BATT_UV_O/1 -> ALM_BATT_UV_st/2
  ALM_BATT_UV_st/1 -> ALM_BATT_UV_D/1
  ALM_BATT_UV_F/1 -> ALM_BATT_UV_D/2
  ALM_BATT_UV_D/1 -> ALM_BATT_UVRon/1
  ALM_BATT_UVRon/1 -> ALM_BATT_UV_S/1
  ALM_BATT_UV_S/1 -> ALM_BATT_UV_1sat/1
  ALM_BATT_UV_1sat/1 -> ALM_BATT_UV_Convert1/1
  ALM_BATT_UV_Convert1/1 -> ALM_BATT_UV_L/1
  ALM_BATT_UV_L/1 -> ALM_BATT_UV_Convert/1
  ALM_BATT_UV_Convert/1 -> output2/1

== system FSAC2021/ROUTING/TO_DCAN/Subsystem/DIAG_BMS_ALARM_RELAY/ALM_BMU_FAIL ==
  ALM_BMU_FAIL : Inport
  ALM_BMU_FAILRon : Rounding  Operator=round
  ALM_BMU_FAIL_1sat : Saturate  UpperLimit=32  LowerLimit=0
  ALM_BMU_FAIL_Convert : DataTypeConversion  OutDataTypeStr=uint8
  ALM_BMU_FAIL_Convert1 : DataTypeConversion  OutDataTypeStr=uint32
  ALM_BMU_FAIL_D : Product  Inputs=*/
  ALM_BMU_FAIL_F : Constant  OutDataTypeStr=single
  ALM_BMU_FAIL_L : simulink/Logic and Bit Operations/Bitwise Operator  logicop=AND  UseBitMask=on  BitMask=32  BitMaskRealWorld=Stored Integer
  ALM_BMU_FAIL_O : Constant  Value=0  OutDataTypeStr=single
  ALM_BMU_FAIL_S : ArithShift  BitShiftNumber=-5
  ALM_BMU_FAIL_sat : Saturate  UpperLimit=1  LowerLimit=0
  ALM_BMU_FAIL_st : Sum  Inputs=+-
  output3 : Outport
  wires:
  ALM_BMU_FAIL/1 -> ALM_BMU_FAIL_sat/1
  ALM_BMU_FAIL_sat/1 -> ALM_BMU_FAIL_st/1
  ALM_BMU_FAIL_O/1 -> ALM_BMU_FAIL_st/2
  ALM_BMU_FAIL_st/1 -> ALM_BMU_FAIL_D/1
  ALM_BMU_FAIL_F/1 -> ALM_BMU_FAIL_D/2
  ALM_BMU_FAIL_D/1 -> ALM_BMU_FAILRon/1
  ALM_BMU_FAILRon/1 -> ALM_BMU_FAIL_S/1
  ALM_BMU_FAIL_S/1 -> ALM_BMU_FAIL_1sat/1
  ALM_BMU_FAIL_1sat/1 -> ALM_BMU_FAIL_Convert1/1
  ALM_BMU_FAIL_Convert1/1 -> ALM_BMU_FAIL_L/1
  ALM_BMU_FAIL_L/1 -> ALM_BMU_FAIL_Convert/1
  ALM_BMU_FAIL_Convert/1 -> output3/1

== system FSAC2021/ROUTING/TO_DCAN/Subsystem/DIAG_BMS_ALARM_RELAY/ALM_BSU_FAULT ==
  ALM_BSU_FAULT : Inport
  ALM_BSU_FAULTRon : Rounding  Operator=round
  ALM_BSU_FAULT_1sat : Saturate  UpperLimit=2  LowerLimit=0
  ALM_BSU_FAULT_Convert : DataTypeConversion  OutDataTypeStr=uint8
  ALM_BSU_FAULT_Convert1 : DataTypeConversion  OutDataTypeStr=uint32
  ALM_BSU_FAULT_D : Product  Inputs=*/
  ALM_BSU_FAULT_F : Constant  OutDataTypeStr=single
  ALM_BSU_FAULT_L : simulink/Logic and Bit Operations/Bitwise Operator  logicop=AND  UseBitMask=on  BitMask=2  BitMaskRealWorld=Stored Integer
  ALM_BSU_FAULT_O : Constant  Value=0  OutDataTypeStr=single
  ALM_BSU_FAULT_S : ArithShift  BitShiftNumber=-1
  ALM_BSU_FAULT_sat : Saturate  UpperLimit=1  LowerLimit=0
  ALM_BSU_FAULT_st : Sum  Inputs=+-
  output3 : Outport
  wires:
  ALM_BSU_FAULT/1 -> ALM_BSU_FAULT_sat/1
  ALM_BSU_FAULT_sat/1 -> ALM_BSU_FAULT_st/1
  ALM_BSU_FAULT_O/1 -> ALM_BSU_FAULT_st/2
  ALM_BSU_FAULT_st/1 -> ALM_BSU_FAULT_D/1
  ALM_BSU_FAULT_F/1 -> ALM_BSU_FAULT_D/2
  ALM_BSU_FAULT_D/1 -> ALM_BSU_FAULTRon/1
  ALM_BSU_FAULTRon/1 -> ALM_BSU_FAULT_S/1
  ALM_BSU_FAULT_S/1 -> ALM_BSU_FAULT_1sat/1
  ALM_BSU_FAULT_1sat/1 -> ALM_BSU_FAULT_Convert1/1
  ALM_BSU_FAULT_Convert1/1 -> ALM_BSU_FAULT_L/1
  ALM_BSU_FAULT_L/1 -> ALM_BSU_FAULT_Convert/1
  ALM_BSU_FAULT_Convert/1 -> output3/1

== system FSAC2021/ROUTING/TO_DCAN/Subsystem/DIAG_BMS_ALARM_RELAY/ALM_BSU_OFFLINE ==
  ALM_BSU_OFFLINE : Inport
  ALM_BSU_OFFLINERon : Rounding  Operator=round
  ALM_BSU_OFFLINE_1sat : Saturate  UpperLimit=1  LowerLimit=0
  ALM_BSU_OFFLINE_Convert : DataTypeConversion  OutDataTypeStr=uint8
  ALM_BSU_OFFLINE_Convert1 : DataTypeConversion  OutDataTypeStr=uint32
  ALM_BSU_OFFLINE_D : Product  Inputs=*/
  ALM_BSU_OFFLINE_F : Constant  OutDataTypeStr=single
  ALM_BSU_OFFLINE_L : simulink/Logic and Bit Operations/Bitwise Operator  logicop=AND  UseBitMask=on  BitMask=1  BitMaskRealWorld=Stored Integer
  ALM_BSU_OFFLINE_O : Constant  Value=0  OutDataTypeStr=single
  ALM_BSU_OFFLINE_S : ArithShift
  ALM_BSU_OFFLINE_sat : Saturate  UpperLimit=1  LowerLimit=0
  ALM_BSU_OFFLINE_st : Sum  Inputs=+-
  output3 : Outport
  wires:
  ALM_BSU_OFFLINE/1 -> ALM_BSU_OFFLINE_sat/1
  ALM_BSU_OFFLINE_sat/1 -> ALM_BSU_OFFLINE_st/1
  ALM_BSU_OFFLINE_O/1 -> ALM_BSU_OFFLINE_st/2
  ALM_BSU_OFFLINE_st/1 -> ALM_BSU_OFFLINE_D/1
  ALM_BSU_OFFLINE_F/1 -> ALM_BSU_OFFLINE_D/2
  ALM_BSU_OFFLINE_D/1 -> ALM_BSU_OFFLINERon/1
  ALM_BSU_OFFLINERon/1 -> ALM_BSU_OFFLINE_S/1
  ALM_BSU_OFFLINE_S/1 -> ALM_BSU_OFFLINE_1sat/1
  ALM_BSU_OFFLINE_1sat/1 -> ALM_BSU_OFFLINE_Convert1/1
  ALM_BSU_OFFLINE_Convert1/1 -> ALM_BSU_OFFLINE_L/1
  ALM_BSU_OFFLINE_L/1 -> ALM_BSU_OFFLINE_Convert/1
  ALM_BSU_OFFLINE_Convert/1 -> output3/1

== system FSAC2021/ROUTING/TO_DCAN/Subsystem/DIAG_BMS_ALARM_RELAY/ALM_CELL_IBK ==
  ALM_CELL_IBK : Inport
  ALM_CELL_IBKRon : Rounding  Operator=round
  ALM_CELL_IBK_1sat : Saturate  UpperLimit=16  LowerLimit=0
  ALM_CELL_IBK_Convert : DataTypeConversion  OutDataTypeStr=uint8
  ALM_CELL_IBK_Convert1 : DataTypeConversion  OutDataTypeStr=uint32
  ALM_CELL_IBK_D : Product  Inputs=*/
  ALM_CELL_IBK_F : Constant  OutDataTypeStr=single
  ALM_CELL_IBK_L : simulink/Logic and Bit Operations/Bitwise Operator  logicop=AND  UseBitMask=on  BitMask=16  BitMaskRealWorld=Stored Integer
  ALM_CELL_IBK_O : Constant  Value=0  OutDataTypeStr=single
  ALM_CELL_IBK_S : ArithShift  BitShiftNumber=-4
  ALM_CELL_IBK_sat : Saturate  UpperLimit=1  LowerLimit=0
  ALM_CELL_IBK_st : Sum  Inputs=+-
  output1 : Outport
  wires:
  ALM_CELL_IBK/1 -> ALM_CELL_IBK_sat/1
  ALM_CELL_IBK_sat/1 -> ALM_CELL_IBK_st/1
  ALM_CELL_IBK_O/1 -> ALM_CELL_IBK_st/2
  ALM_CELL_IBK_st/1 -> ALM_CELL_IBK_D/1
  ALM_CELL_IBK_F/1 -> ALM_CELL_IBK_D/2
  ALM_CELL_IBK_D/1 -> ALM_CELL_IBKRon/1
  ALM_CELL_IBKRon/1 -> ALM_CELL_IBK_S/1
  ALM_CELL_IBK_S/1 -> ALM_CELL_IBK_1sat/1
  ALM_CELL_IBK_1sat/1 -> ALM_CELL_IBK_Convert1/1
  ALM_CELL_IBK_Convert1/1 -> ALM_CELL_IBK_L/1
  ALM_CELL_IBK_L/1 -> ALM_CELL_IBK_Convert/1
  ALM_CELL_IBK_Convert/1 -> output1/1

== system FSAC2021/ROUTING/TO_DCAN/Subsystem/DIAG_BMS_ALARM_RELAY/ALM_CELL_OT ==
  ALM_CELL_OT : Inport
  ALM_CELL_OTRon : Rounding  Operator=round
  ALM_CELL_OT_1sat : Saturate  UpperLimit=4  LowerLimit=0
  ALM_CELL_OT_Convert : DataTypeConversion  OutDataTypeStr=uint8
  ALM_CELL_OT_Convert1 : DataTypeConversion  OutDataTypeStr=uint32
  ALM_CELL_OT_D : Product  Inputs=*/
  ALM_CELL_OT_F : Constant  OutDataTypeStr=single
  ALM_CELL_OT_L : simulink/Logic and Bit Operations/Bitwise Operator  logicop=AND  UseBitMask=on  BitMask=4  BitMaskRealWorld=Stored Integer
  ALM_CELL_OT_O : Constant  Value=0  OutDataTypeStr=single
  ALM_CELL_OT_S : ArithShift  BitShiftNumber=-2
  ALM_CELL_OT_sat : Saturate  UpperLimit=1  LowerLimit=0
  ALM_CELL_OT_st : Sum  Inputs=+-
  output1 : Outport
  wires:
  ALM_CELL_OT/1 -> ALM_CELL_OT_sat/1
  ALM_CELL_OT_sat/1 -> ALM_CELL_OT_st/1
  ALM_CELL_OT_O/1 -> ALM_CELL_OT_st/2
  ALM_CELL_OT_st/1 -> ALM_CELL_OT_D/1
  ALM_CELL_OT_F/1 -> ALM_CELL_OT_D/2
  ALM_CELL_OT_D/1 -> ALM_CELL_OTRon/1
  ALM_CELL_OTRon/1 -> ALM_CELL_OT_S/1
  ALM_CELL_OT_S/1 -> ALM_CELL_OT_1sat/1
  ALM_CELL_OT_1sat/1 -> ALM_CELL_OT_Convert1/1
  ALM_CELL_OT_Convert1/1 -> ALM_CELL_OT_L/1
  ALM_CELL_OT_L/1 -> ALM_CELL_OT_Convert/1
  ALM_CELL_OT_Convert/1 -> output1/1

== system FSAC2021/ROUTING/TO_DCAN/Subsystem/DIAG_BMS_ALARM_RELAY/ALM_CELL_OV ==
  ALM_CELL_OV : Inport
  ALM_CELL_OVRon : Rounding  Operator=round
  ALM_CELL_OV_1sat : Saturate  UpperLimit=1  LowerLimit=0
  ALM_CELL_OV_Convert : DataTypeConversion  OutDataTypeStr=uint8
  ALM_CELL_OV_Convert1 : DataTypeConversion  OutDataTypeStr=uint32
  ALM_CELL_OV_D : Product  Inputs=*/
  ALM_CELL_OV_F : Constant  OutDataTypeStr=single
  ALM_CELL_OV_L : simulink/Logic and Bit Operations/Bitwise Operator  logicop=AND  UseBitMask=on  BitMask=1  BitMaskRealWorld=Stored Integer
  ALM_CELL_OV_O : Constant  Value=0  OutDataTypeStr=single
  ALM_CELL_OV_S : ArithShift
  ALM_CELL_OV_sat : Saturate  UpperLimit=1  LowerLimit=0
  ALM_CELL_OV_st : Sum  Inputs=+-
  output1 : Outport
  wires:
  ALM_CELL_OV/1 -> ALM_CELL_OV_sat/1
  ALM_CELL_OV_sat/1 -> ALM_CELL_OV_st/1
  ALM_CELL_OV_O/1 -> ALM_CELL_OV_st/2
  ALM_CELL_OV_st/1 -> ALM_CELL_OV_D/1
  ALM_CELL_OV_F/1 -> ALM_CELL_OV_D/2
  ALM_CELL_OV_D/1 -> ALM_CELL_OVRon/1
  ALM_CELL_OVRon/1 -> ALM_CELL_OV_S/1
  ALM_CELL_OV_S/1 -> ALM_CELL_OV_1sat/1
  ALM_CELL_OV_1sat/1 -> ALM_CELL_OV_Convert1/1
  ALM_CELL_OV_Convert1/1 -> ALM_CELL_OV_L/1
  ALM_CELL_OV_L/1 -> ALM_CELL_OV_Convert/1
  ALM_CELL_OV_Convert/1 -> output1/1

== system FSAC2021/ROUTING/TO_DCAN/Subsystem/DIAG_BMS_ALARM_RELAY/ALM_CELL_TBK ==
  ALM_CELL_TBK : Inport
  ALM_CELL_TBKRon : Rounding  Operator=round
  ALM_CELL_TBK_1sat : Saturate  UpperLimit=32  LowerLimit=0
  ALM_CELL_TBK_Convert : DataTypeConversion  OutDataTypeStr=uint8
  ALM_CELL_TBK_Convert1 : DataTypeConversion  OutDataTypeStr=uint32
  ALM_CELL_TBK_D : Product  Inputs=*/
  ALM_CELL_TBK_F : Constant  OutDataTypeStr=single
  ALM_CELL_TBK_L : simulink/Logic and Bit Operations/Bitwise Operator  logicop=AND  UseBitMask=on  BitMask=32  BitMaskRealWorld=Stored Integer
  ALM_CELL_TBK_O : Constant  Value=0  OutDataTypeStr=single
  ALM_CELL_TBK_S : ArithShift  BitShiftNumber=-5
  ALM_CELL_TBK_sat : Saturate  UpperLimit=1  LowerLimit=0
  ALM_CELL_TBK_st : Sum  Inputs=+-
  output1 : Outport
  wires:
  ALM_CELL_TBK/1 -> ALM_CELL_TBK_sat/1
  ALM_CELL_TBK_sat/1 -> ALM_CELL_TBK_st/1
  ALM_CELL_TBK_O/1 -> ALM_CELL_TBK_st/2
  ALM_CELL_TBK_st/1 -> ALM_CELL_TBK_D/1
  ALM_CELL_TBK_F/1 -> ALM_CELL_TBK_D/2
  ALM_CELL_TBK_D/1 -> ALM_CELL_TBKRon/1
  ALM_CELL_TBKRon/1 -> ALM_CELL_TBK_S/1
  ALM_CELL_TBK_S/1 -> ALM_CELL_TBK_1sat/1
  ALM_CELL_TBK_1sat/1 -> ALM_CELL_TBK_Convert1/1
  ALM_CELL_TBK_Convert1/1 -> ALM_CELL_TBK_L/1
  ALM_CELL_TBK_L/1 -> ALM_CELL_TBK_Convert/1
  ALM_CELL_TBK_Convert/1 -> output1/1

== system FSAC2021/ROUTING/TO_DCAN/Subsystem/DIAG_BMS_ALARM_RELAY/ALM_CELL_UT ==
  ALM_CELL_UT : Inport
  ALM_CELL_UTRon : Rounding  Operator=round
  ALM_CELL_UT_1sat : Saturate  UpperLimit=8  LowerLimit=0
  ALM_CELL_UT_Convert : DataTypeConversion  OutDataTypeStr=uint8
  ALM_CELL_UT_Convert1 : DataTypeConversion  OutDataTypeStr=uint32
  ALM_CELL_UT_D : Product  Inputs=*/
  ALM_CELL_UT_F : Constant  OutDataTypeStr=single
  ALM_CELL_UT_L : simulink/Logic and Bit Operations/Bitwise Operator  logicop=AND  UseBitMask=on  BitMask=8  BitMaskRealWorld=Stored Integer
  ALM_CELL_UT_O : Constant  Value=0  OutDataTypeStr=single
  ALM_CELL_UT_S : ArithShift  BitShiftNumber=-3
  ALM_CELL_UT_sat : Saturate  UpperLimit=1  LowerLimit=0
  ALM_CELL_UT_st : Sum  Inputs=+-
  output1 : Outport
  wires:
  ALM_CELL_UT/1 -> ALM_CELL_UT_sat/1
  ALM_CELL_UT_sat/1 -> ALM_CELL_UT_st/1
  ALM_CELL_UT_O/1 -> ALM_CELL_UT_st/2
  ALM_CELL_UT_st/1 -> ALM_CELL_UT_D/1
  ALM_CELL_UT_F/1 -> ALM_CELL_UT_D/2
  ALM_CELL_UT_D/1 -> ALM_CELL_UTRon/1
  ALM_CELL_UTRon/1 -> ALM_CELL_UT_S/1
  ALM_CELL_UT_S/1 -> ALM_CELL_UT_1sat/1
  ALM_CELL_UT_1sat/1 -> ALM_CELL_UT_Convert1/1
  ALM_CELL_UT_Convert1/1 -> ALM_CELL_UT_L/1
  ALM_CELL_UT_L/1 -> ALM_CELL_UT_Convert/1
  ALM_CELL_UT_Convert/1 -> output1/1

== system FSAC2021/ROUTING/TO_DCAN/Subsystem/DIAG_BMS_ALARM_RELAY/ALM_CELL_UV ==
  ALM_CELL_UV : Inport
  ALM_CELL_UVRon : Rounding  Operator=round
  ALM_CELL_UV_1sat : Saturate  UpperLimit=2  LowerLimit=0
  ALM_CELL_UV_Convert : DataTypeConversion  OutDataTypeStr=uint8
  ALM_CELL_UV_Convert1 : DataTypeConversion  OutDataTypeStr=uint32
  ALM_CELL_UV_D : Product  Inputs=*/
  ALM_CELL_UV_F : Constant  OutDataTypeStr=single
  ALM_CELL_UV_L : simulink/Logic and Bit Operations/Bitwise Operator  logicop=AND  UseBitMask=on  BitMask=2  BitMaskRealWorld=Stored Integer
  ALM_CELL_UV_O : Constant  Value=0  OutDataTypeStr=single
  ALM_CELL_UV_S : ArithShift  BitShiftNumber=-1
  ALM_CELL_UV_sat : Saturate  UpperLimit=1  LowerLimit=0
  ALM_CELL_UV_st : Sum  Inputs=+-
  output1 : Outport
  wires:
  ALM_CELL_UV/1 -> ALM_CELL_UV_sat/1
  ALM_CELL_UV_sat/1 -> ALM_CELL_UV_st/1
  ALM_CELL_UV_O/1 -> ALM_CELL_UV_st/2
  ALM_CELL_UV_st/1 -> ALM_CELL_UV_D/1
  ALM_CELL_UV_F/1 -> ALM_CELL_UV_D/2
  ALM_CELL_UV_D/1 -> ALM_CELL_UVRon/1
  ALM_CELL_UVRon/1 -> ALM_CELL_UV_S/1
  ALM_CELL_UV_S/1 -> ALM_CELL_UV_1sat/1
  ALM_CELL_UV_1sat/1 -> ALM_CELL_UV_Convert1/1
  ALM_CELL_UV_Convert1/1 -> ALM_CELL_UV_L/1
  ALM_CELL_UV_L/1 -> ALM_CELL_UV_Convert/1
  ALM_CELL_UV_Convert/1 -> output1/1

== system FSAC2021/ROUTING/TO_DCAN/Subsystem/DIAG_BMS_ALARM_RELAY/ALM_CHRG_OCS ==
  ALM_CHRG_OCS : Inport
  ALM_CHRG_OCSRon : Rounding  Operator=round
  ALM_CHRG_OCS_1sat : Saturate  UpperLimit=16  LowerLimit=0
  ALM_CHRG_OCS_Convert : DataTypeConversion  OutDataTypeStr=uint8
  ALM_CHRG_OCS_Convert1 : DataTypeConversion  OutDataTypeStr=uint32
  ALM_CHRG_OCS_D : Product  Inputs=*/
  ALM_CHRG_OCS_F : Constant  OutDataTypeStr=single
  ALM_CHRG_OCS_L : simulink/Logic and Bit Operations/Bitwise Operator  logicop=AND  UseBitMask=on  BitMask=16  BitMaskRealWorld=Stored Integer
  ALM_CHRG_OCS_O : Constant  Value=0  OutDataTypeStr=single
  ALM_CHRG_OCS_S : ArithShift  BitShiftNumber=-4
  ALM_CHRG_OCS_sat : Saturate  UpperLimit=1  LowerLimit=0
  ALM_CHRG_OCS_st : Sum  Inputs=+-
  output2 : Outport
  wires:
  ALM_CHRG_OCS/1 -> ALM_CHRG_OCS_sat/1
  ALM_CHRG_OCS_sat/1 -> ALM_CHRG_OCS_st/1
  ALM_CHRG_OCS_O/1 -> ALM_CHRG_OCS_st/2
  ALM_CHRG_OCS_st/1 -> ALM_CHRG_OCS_D/1
  ALM_CHRG_OCS_F/1 -> ALM_CHRG_OCS_D/2
  ALM_CHRG_OCS_D/1 -> ALM_CHRG_OCSRon/1
  ALM_CHRG_OCSRon/1 -> ALM_CHRG_OCS_S/1
  ALM_CHRG_OCS_S/1 -> ALM_CHRG_OCS_1sat/1
  ALM_CHRG_OCS_1sat/1 -> ALM_CHRG_OCS_Convert1/1
  ALM_CHRG_OCS_Convert1/1 -> ALM_CHRG_OCS_L/1
  ALM_CHRG_OCS_L/1 -> ALM_CHRG_OCS_Convert/1
  ALM_CHRG_OCS_Convert/1 -> output2/1

== system FSAC2021/ROUTING/TO_DCAN/Subsystem/DIAG_BMS_ALARM_RELAY/ALM_CHRG_OCT ==
  ALM_CHRG_OCT : Inport
  ALM_CHRG_OCTRon : Rounding  Operator=round
  ALM_CHRG_OCT_1sat : Saturate  UpperLimit=64  LowerLimit=0
  ALM_CHRG_OCT_Convert : DataTypeConversion  OutDataTypeStr=uint8
  ALM_CHRG_OCT_Convert1 : DataTypeConversion  OutDataTypeStr=uint32
  ALM_CHRG_OCT_D : Product  Inputs=*/
  ALM_CHRG_OCT_F : Constant  OutDataTypeStr=single
  ALM_CHRG_OCT_L : simulink/Logic and Bit Operations/Bitwise Operator  logicop=AND  UseBitMask=on  BitMask=64  BitMaskRealWorld=Stored Integer
  ALM_CHRG_OCT_O : Constant  Value=0  OutDataTypeStr=single
  ALM_CHRG_OCT_S : ArithShift  BitShiftNumber=-6
  ALM_CHRG_OCT_sat : Saturate  UpperLimit=1  LowerLimit=0
  ALM_CHRG_OCT_st : Sum  Inputs=+-
  output2 : Outport
  wires:
  ALM_CHRG_OCT/1 -> ALM_CHRG_OCT_sat/1
  ALM_CHRG_OCT_sat/1 -> ALM_CHRG_OCT_st/1
  ALM_CHRG_OCT_O/1 -> ALM_CHRG_OCT_st/2
  ALM_CHRG_OCT_st/1 -> ALM_CHRG_OCT_D/1
  ALM_CHRG_OCT_F/1 -> ALM_CHRG_OCT_D/2
  ALM_CHRG_OCT_D/1 -> ALM_CHRG_OCTRon/1
  ALM_CHRG_OCTRon/1 -> ALM_CHRG_OCT_S/1
  ALM_CHRG_OCT_S/1 -> ALM_CHRG_OCT_1sat/1
  ALM_CHRG_OCT_1sat/1 -> ALM_CHRG_OCT_Convert1/1
  ALM_CHRG_OCT_Convert1/1 -> ALM_CHRG_OCT_L/1
  ALM_CHRG_OCT_L/1 -> ALM_CHRG_OCT_Convert/1
  ALM_CHRG_OCT_Convert/1 -> output2/1
